simulink model "GroundRelayOC"  (R2025a)
settings: Solver=ode23tb  StartTime=0.0  StopTime=1  RelTol=1e-3  EnableMultiTasking=on
libraries: spsThreePhaseSeriesRLCLoadLib x5, spsDistributedParametersLineLib x5, spsThreePhaseVIMeasurementLib x2, spsRMSLib x1, spsThreePhaseBreakerLib x1, spsThreePhaseFaultLib x1, spsThreePhaseSourceLib x1, spspowerguiLib x1
settings Model: Creator=Rodney Tan  LastModifiedBy=Sanny
settings SolverCC: AlgebraicLoopSolver=TrustRegion
settings DataIOCC: LimitDataPoints=on  SaveFormat=Array  ReturnWorkspaceOutputs=off
settings OptimizationCC: LifeSpan=inf
settings DebuggingCC: UnconnectedInputMsg=warning  UnconnectedOutputMsg=warning  UnconnectedLineMsg=warning  SFUnexpectedBacktrackingDiag=warning  SFNoUnconditionalDefaultTransitionDiag=warning  SFExecutionAtInitializationDiag=none  ArithmeticOperatorsInVariantConditions=warning
settings HardwareCC: ProdBitPerPointer=32.0  ProdBitPerSizeT=32.0  ProdBitPerPtrDiffT=32.0  ProdLargestAtomicFloat=None  ProdIntDivRoundTo=Undefined  ProdEndianess=Unspecified  ProdWordSize=32.0  ProdHWDeviceType=32-bit Generic
settings ModelReferenceCC: EnableRefExpFcnMdlSchedulingChecks=on  PropagateSignalLabelsOutOfModel=off
settings SFSimCC: SimUseLocalCustomCode=off  CustomCodeUndefinedFunction=UseInterfaceOnly
settings RTWCC: RTWUseLocalCustomCode=off  GPUComputeCapability=3.5
settings CodeAppCC: StateflowObjectComments=on
settings GRTTargetCC: TargetLangStandard=C89/C90 (ANSI)
settings ConfigComp: CovMetricSettings=dw  CovSaveCumulativeToWorkspaceVar=on  CovSaveSingleToWorkspaceVar=on  CovExternalEMLEnable=off
settings SimscapeCC: SimscapeNormalizeSystem=off

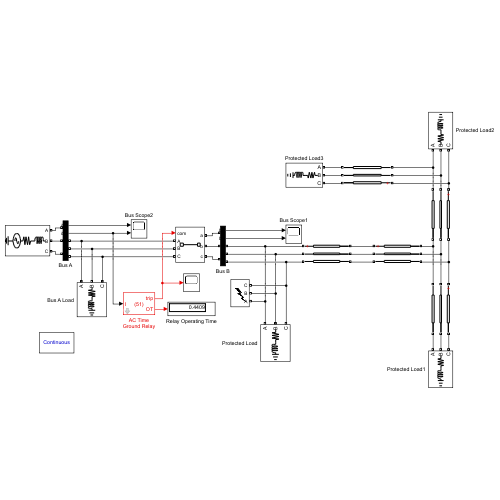
[thumbnail: Simulink's stored preview of the top-level diagram]
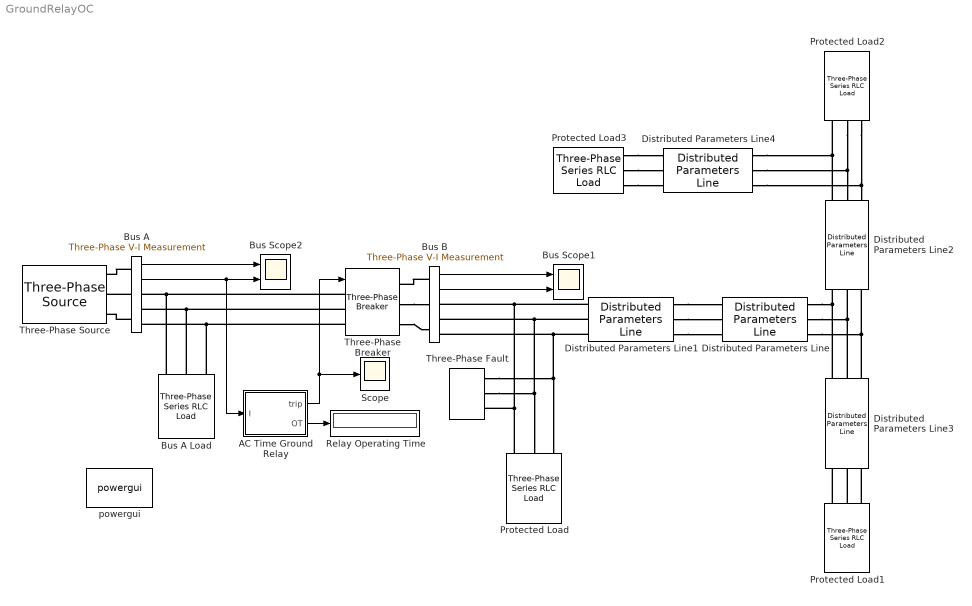
== system GroundRelayOC ==
  AC Time Ground Relay : Subsystem  mask(AC Time Ground Relay Block){tcpopup=IEC Standard Inverse, k=0.14, alpha=0.02, B=0, PS=100%, TMS=0.1, TDS=0.1, CTpri=300, CTsec=5, Freq=50, RMSInit=0}
      mask prompts: tcpopup "Trip Characteristic"; PS "Plug Setting (PS) / Low-set (I >)"; TMS "Time Multiplier Setting (TMS)"; TDS "Time Delay Setting (TDS) in sec"; CTpri "Current Transformer Primary (A)"; CTsec "Current Transformer Secondary (A)"; Freq "Fundamental frequency (Hz):"; RMSInit "Initial RMS value:"
      mask help:
      | AC Time Ground Relay Block developed
      |
      | AC Time Ground  Relay (ANSI/IEEE C37.2 device number 51) that operates when the current exceeds a predetermined value.
      |
      | This relay operates with either a Definite Minimum Time (DMT) or Inverse Definite Minimum Time (IDMT) characteristic.
      |
      | This relay support both IEC 60255 Standard and IEEE Standard C37.112-1996 IDMT trip characteristic.
      mask Help:
      | <b><u>Block Setting</u></b>
      | <b>Trip Characteristic</b>
      | Relay operation mode selection of Definite Minimum Time (DMT), IEC 60255 Standard or IEEE Standard C37.112-1996 Inverse Definite Minimum Time (IDMT).
      | 
      | <b>Plug-Setting(PS) / Low-set (I >)</b>
      | Specify relay pick-up current based on current transformer rating ranging from 25% to 200% with 25% step interval.
      | 
      | <b>Time Multiplier Setting (TMS)</b>
      | Specify time delay multiplier ranging from 0.05 to 1.0 for IDMT relay operation. This setting will be disabled DMT relay operation mode.
      | 
      | <b>Plot Curve Button</b>
      | Plot current Inverse Definite Minimum Time trip curve.
      | 
      | <b>Time Delay Setting (TDS)</b>
      | Specify time delay ranging from 0.05sec to 99sec for Definite Minimum Time relay operation. This setting will be disabled in IDMT relay operation mode.
      | 
      | <b>Current Transformer Primary (A)</b>
      | Specify current transformer primary in Ampere.
      | 
      | <b>Current Transformer Secondary (A)</b>
      | Specify current transformer secondary in Ampere.
      | 
      | <b>Fundamental Frequency (Hz)</b>
      | Specify the RMS current measurement fundamental frequency, in hertz, of the input signal.
      | 
      | <b>Initial RMS Value</b>
      | Specify the RMS current measurement initial RMS value of the output signal.
      | 
      | <b><u>Block Input Output</u></b>
      | <b>I</b>
      | Current input to the AC time overcurrent relay
      | 
      | <b>trip</b>
      | Trip control signal output (1-0), commonly connected to circuit breaker
      | 
      | <b>OT</b>
      | Relay operating time output
      mask TypeOptions tcpopup: Definite Minimum Time | IEC Standard Inverse | IEC Very Inverse | IEC Long Time Inverse | IEC Extremely Inverse | IEC Ultra Inverse | IEEE Moderately Inverse | IEEE Very Inverse | IEEE Extremely Inverse
      mask Callback tcpopup:
      | switch(get_param(gcb,'tcpopup'))
      |     case 'IEC Standard Inverse'
      |         set_param(gcb,'k','0.14');
      |         set_param(gcb,'alpha','0.02');
      |         set_param(gcb,'B','0');
      |         set_param(gcb,'MaskEnables',{'on','off','off','off',...
      |                   'on','on','off','on','on','on','on'});
      |     case 'IEC Very Inverse'
      |         set_param(gcb,'k','13.5');
      |         set_param(gcb,'alpha','1');
      |         set_param(gcb,'B','0');
      |         set_param(gcb,'MaskEnables',{'on','off','off','off',...
      |                   'on','on','off','on','on','on','on'});
      |     case 'IEC Long Time Inverse'
      |         set_param(gcb,'k','120');
      |         set_param(gcb,'alpha','1');
      |         set_param(gcb,'B','0');
      |         set_param(gcb,'MaskEnables',{'on','off','off','off',...
      |                   'on','on','off','on','on','on','on'});
      |     case 'IEC Extremely Inverse'
      |         set_param(gcb,'k','80');
      |         set_param(gcb,'alpha','2');
      |         set_param(gcb,'B','0');
      |         set_param(gcb,'MaskEnables',{'on','off','off','off',...
      |                   'on','on','off','on','on','on','on'});
      |     case 'IEC Ultra Inverse'
      |         set_param(gcb,'k','315.2');
      |         set_param(gcb,'alpha','2.5');
      |         set_param(gcb,'B','0');
      |         set_param(gcb,'MaskEnables',{'on','off','off','off',...
      |                   'on','on','off','on','on','on','on'});
      |     case 'IEEE Moderately Inverse'
      |         set_param(gcb,'k','0.0515');
      |         set_param(gcb,'alpha','0.02');
      |         set_param(gcb,'B','0.114');
      |         set_param(gcb,'MaskEnables',{'on','off','off','off',...
      |                   'on','on','off','on','on','on','on'});
      |     case 'IEEE Very Inverse'
      |         set_param(gcb,'k','19.61');
      |         set_param(gcb,'alpha','2');
      |         set_param(gcb,'B','0.491');
      |         set_param(gcb,'MaskEnables',{'on','off','off','off',...
      |                   'on','on','off','on','on','on','on'});
      |     case 'IEEE Extremely Inverse'
      |         set_param(gcb,'k','28.2');
      |         set_param(gcb,'alpha','2');
      |         set_param(gcb,'B','0.1217');
      |         set_param(gcb,'MaskEnables',{'on','off','off','off',...
      |                   'on','on','off','on','on','on','on'});
      |     otherwise
      |         set_param(gcb,'k','0');
      |         set_param(gcb,'MaskEnables',{'on','off','off','off',...
      |                   'on','off','on','on','on','on','on'});
      | end
      mask TypeOptions PS: 25% | 50% | 75% | 100% | 125% | 150% | 175% | 200%
      mask TypeOptions TMS: 0.05 | 0.1 | 0.15 | 0.2 | 0.25 | 0.3 | 0.35 | 0.4 | 0.45 | 0.5 | 0.55 | 0.6 | 0.65 | 0.7 | 0.75 | 0.8 | 0.85 | 0.9 | 0.95 | 1.0
      mask Callback TDS:
      | TDS = str2double(get_param(gcb,'TDS'));
      | if (TDS > 99)||(TDS < 0.05)||isnan(TDS)
      |     msgbox('TDS must be in the range of 0.05-99 sec',...
      |     'Invalid Value !','error');
      |     set_param(gcb,'TDS','0.1');
      | end
      mask TypeOptions Freq: Irms/Freq
      mask TypeOptions RMSInit: Irms/RMSInit
      mask DialogControl Container2 Prompt: Relay Setting
      mask DialogControl plotbutton Prompt: Plot Curve
      mask DialogControl plotbutton Callback:
      | % Plotting IDMT Curve
      | TMS = str2num(get_param(gcb,'TMS'));
      | k = str2num(get_param(gcb,'k'));
      | alpha = str2num(get_param(gcb,'alpha'));
      | B = str2num(get_param(gcb,'B'));
      | I = 1:20;
      | td = ((k./((I.^alpha)-1))+B)*TMS;
      | loglog(td);
      | set(gcf, 'Position', [200 150 300 500]);
      | switch(get_param(gcb,'tcpopup'))
      |     case 'IEC Standard Inverse'
      |         title('IEC Standard Inverse');
      |         set(gca, 'YTick', (1:10));
      |         ylim([0.1 10]);
      |     case 'IEC Very Inverse'
      |         title('IEC Very Inverse');
      |         set(gca, 'YTick', (1:2:15));
      |         ylim([0.01 15]);
      |     case 'IEC Long Time Inverse'
      |         title('IEC Long Time Inverse');
      |         set(gca, 'YTick', (0:20:120));
      |         ylim([0.1 120]);
      |     case 'IEC Extremely Inverse'
      |         title('IEC Extremely Inverse');
      |         set(gca, 'YTick', (0:5:30));
      |         ylim([0.01 30]);
      |     case 'IEC Ultra Inverse'
      |         title('IEC Ultra Inverse');
      |         set(gca, 'YTick', (0:20:100));
      |         ylim([0.01 100]);
      |     case 'IEEE Moderately Inverse'
      |         title('IEEE Moderately Inverse');
      |         set(gca, 'YTick', (1:5));
      |         ylim([0.01 5]);
      |     case 'IEEE Very Inverse'
      |         title('IEEE Very Inverse');
      |         set(gca, 'YTick', (1:10));
      |         ylim([0.01 10]);
      |     case 'IEEE Extremely Inverse'
      |         title('IEEE Extremely Inverse');
      |         set(gca, 'YTick', (1:10));
      |         ylim([0.01 10]);
      | end
      | 
      | set(gca, 'XTick', [1:10 20]);
      | xlim([1 30]);
      | xlabel('Current (Multiples of Plug Setting)');
      | ylabel('Operating Time (sec)');
      | grid on;
      mask DialogControl Container3 Prompt: Current Transformer Setting
      mask DialogControl RMS Prompt: RMS Current Measurement
      mask Display:
      | disp('(51)');
      | port_label('input', 1, 'I');
      | port_label('output', 1, 'trip');
      | port_label('output', 2, 'OT');
  Bus A : spsThreePhaseVIMeasurementLib/Three-Phase V-I Measurement  VoltageMeasurement=phase-to-ground  SetLabelV=off  LabelV=Vabc  Vpu=off  VpuLL=off  CurrentMeasurement=yes  SetLabelI=off  LabelI=Iabc  Ipu=off  Pbase=100e6  Vbase=500e3  OutputType=Complex  PhasorSimulation=off  PSBequivalent=0
  Bus A Load : spsThreePhaseSeriesRLCLoadLib/Three-Phase Series RLC Load  LConnTagsString=A|B|C  Configuration=Y (grounded)  NominalVoltage=400  Vabc=[1e3 1e3 1e3]  Vabcp=[1e3 1e3 1e3]  NominalFrequency=50  UnbalancedPower=off  ActivePower=100e3  InductivePower=1000  CapacitivePower=0  Pabc=[10e3 9e3 11e3]  QLabc=[100 90 110]  QCabc=[100 90 110]  Pabcp=[10e3 9e3 11e3]  QLabcp=[100 90 110]  QCabcp=[100 90 110]  Measurements=None  LoadType=constant Z
  Bus B : spsThreePhaseVIMeasurementLib/Three-Phase V-I Measurement  VoltageMeasurement=phase-to-ground  SetLabelV=off  LabelV=Vabc  Vpu=off  VpuLL=off  CurrentMeasurement=yes  SetLabelI=off  LabelI=Iabc  Ipu=off  Pbase=100e6  Vbase=500e3  OutputType=Complex  PhasorSimulation=off  PSBequivalent=0
  Bus Scope1 : Scope  NumInputPorts=2
      settings: Title=Bus B Current Profile  ShowGrid=off  ActiveDisplayYMinimum=-2533.58175  ActiveDisplayYMaximum=3369.6826  YLabel=Current (A)  DataLoggingSaveFormat=Array
  Bus Scope2 : Scope  NumInputPorts=2
      settings: Title=Bus A Current Profile  ShowGrid=off  ActiveDisplayYMinimum=-3316.7768762510213  ActiveDisplayYMaximum=3723.0047575859285  YLabel=Current (A)  DataLoggingSaveFormat=Array
  Distributed Parameters Line : spsDistributedParametersLineLib/Distributed Parameters Line  Phases=3  Length=100  Frequency=60  Resistance=[0.01273 0.3864]  Inductance="[0.9337e-3  4.1264e-3]"  Capacitance=[12.74e-9 7.751e-9]  x1=[1.91730079564317e-11 400.864028866089 400.864028866057;314.159265358979 314.159265358979 314.159265358979;-1.26095069546775 0.22104226848999 -1.34975405830491]  x2=[2.10404277961572e-11 418.154854663515 418.154854663482;314.159265358979 314.159265358979 314.159265358979;-1.25793304118418 0.218562240810716 -1.35223408598418]  x3=[3.3168484674381e-14 1.61146629060892 1.6114662906088;314.159265358979 314.159265358979 314.159265358979;-1.67750735657674 -0.207558438130243 -1.77835476492514]  x4=[2.86533303244721e-14 1.6281634973106 1.62816349731047;314.159265358979 314.159265358979 314.159265358979;-0.811737549604632 0.534619710597266 -1.03617661619763]  x5=0.000565541566995742  V1=[1.917e-11 400.9 400.9;314.2 314.2 314.2;-1.261 0.221 -1.35]  V2=[2.104e-11 418.2 418.2;314.2 314.2 314.2;-1.258 0.2186 -1.352]  I1=[3.317e-14 1.611 1.611;314.2 314.2 314.2;-1.678 -0.2076 -1.778]  I2=[2.865e-14 1.628 1.628;314.2 314.2 314.2;-0.8117 0.5346 -1.036]  nHarmo=1  Measurements=None  Decoupling=off  VsMag0=0  VrMag0=0  VsAngle0=0  VrAngle0=0  IsMag0=0  IrMag0=0  IsAngle0=0  IrAngle0=0
      settings: LibrarySourceBlock=sps_lib/Power Grid Elements/Distributed Parameters Line
  Distributed Parameters Line1 : spsDistributedParametersLineLib/Distributed Parameters Line  Phases=3  Length=100  Frequency=60  Resistance=[0.01273 0.3864]  Inductance="[0.9337e-3  4.1264e-3]"  Capacitance=[12.74e-9 7.751e-9]  x1=[1.66634921443281e-11 378.874881999354 378.874881999324;314.159265358979 314.159265358979 314.159265358979;-1.25735531670556 0.22431743741207 -1.34647888938283]  x2=[1.91981231328159e-11 400.864028866089 400.864028866057;314.159265358979 314.159265358979 314.159265358979;-1.26164418272018 0.22104226848999 -1.34975405830491]  x3=[3.2858812901172e-14 1.61004045973489 1.61004045973477;314.159265358979 314.159265358979 314.159265358979;-1.86057715853467 -0.314042437625186 -1.88483876442008]  x4=[2.74177794533837e-14 1.62934933429943 1.62934933429929;314.159265358979 314.159265358979 314.159265358979;-0.630736116597079 0.644633634719405 -0.926162692075487]  x5=0.000565541566995742  V1=[1.666e-11 378.9 378.9;314.2 314.2 314.2;-1.257 0.2243 -1.346]  V2=[1.92e-11 400.9 400.9;314.2 314.2 314.2;-1.262 0.221 -1.35]  I1=[3.286e-14 1.61 1.61;314.2 314.2 314.2;-1.861 -0.314 -1.885]  I2=[2.742e-14 1.629 1.629;314.2 314.2 314.2;-0.6307 0.6446 -0.9262]  nHarmo=1  Measurements=None  Decoupling=off  VsMag0=0  VrMag0=0  VsAngle0=0  VrAngle0=0  IsMag0=0  IrMag0=0  IsAngle0=0  IrAngle0=0
      settings: LibrarySourceBlock=sps_lib/Power Grid Elements/Distributed Parameters Line
  Distributed Parameters Line2 : spsDistributedParametersLineLib/Distributed Parameters Line  Phases=3  Length=100  Frequency=60  Resistance=[0.01273 0.3864]  Inductance="[0.9337e-3  4.1264e-3]"  Capacitance=[12.74e-9 7.751e-9]  x1=[2.2104307302334e-11 425.635026191159 425.635026191177;314.159265358979 314.159265358979 314.159265358979;-1.27734341959448 1.264607271327 2.83540359812197]  x2=[2.10312439975579e-11 418.15485466349 418.154854663507;314.159265358979 314.159265358979 314.159265358979;-1.2573167080909 1.26575979200728 2.83655611880225]  x3=[3.12380835243649e-14 1.58125065905922 1.58125065905928;314.159265358979 314.159265358979 314.159265358979;-1.05804899780135 1.37238132652106 2.94317765331603]  x4=[3.00220202002779e-14 1.57045481453233 1.5704548145324;314.159265358979 314.159265358979 314.159265358979;-1.58568603341573 1.04837602697857 2.61917235377353]  x5=0.000565541566995742  V1=[2.21e-11 425.6 425.6;314.2 314.2 314.2;-1.277 1.265 2.835]  V2=[2.103e-11 418.2 418.2;314.2 314.2 314.2;-1.257 1.266 2.837]  I1=[3.124e-14 1.581 1.581;314.2 314.2 314.2;-1.058 1.372 2.943]  I2=[3.002e-14 1.57 1.57;314.2 314.2 314.2;-1.586 1.048 2.619]  nHarmo=1  Measurements=None  Decoupling=off  VsMag0=0  VrMag0=0  VsAngle0=0  VrAngle0=0  IsMag0=0  IrMag0=0  IsAngle0=0  IrAngle0=0
      settings: LibrarySourceBlock=sps_lib/Power Grid Elements/Distributed Parameters Line
  Distributed Parameters Line3 : spsDistributedParametersLineLib/Distributed Parameters Line  Phases=3  Length=100  Frequency=60  Resistance=[0.01273 0.3864]  Inductance="[0.9337e-3  4.1264e-3]"  Capacitance=[12.74e-9 7.751e-9]  x1=[2.10187140598747e-11 418.15485466349 418.154854663507;314.159265358979 314.159265358979 314.159265358979;-1.25699782996798 1.26575979200728 2.83655611880225]  x2=[2.12460785323591e-11 420.61040635086 420.610406350877;314.159265358979 314.159265358979 314.159265358979;-1.25968948203942 1.2653207935263 2.83611712032126]  x3=[2.989042365455e-14 1.54558853383228 1.54558853383234;314.159265358979 314.159265358979 314.159265358979;-1.39382361404444 1.15726490876129 2.72806123555627]  x4=[2.93775944398719e-14 1.55083211138511 1.55083211138517;314.159265358979 314.159265358979 314.159265358979;-1.27041654471723 1.26515168163053 2.83594800842548]  x5=0.000565541566995742  V1=[2.102e-11 418.2 418.2;314.2 314.2 314.2;-1.257 1.266 2.837]  V2=[2.125e-11 420.6 420.6;314.2 314.2 314.2;-1.26 1.265 2.836]  I1=[2.989e-14 1.546 1.546;314.2 314.2 314.2;-1.394 1.157 2.728]  I2=[2.938e-14 1.551 1.551;314.2 314.2 314.2;-1.27 1.265 2.836]  nHarmo=1  Measurements=None  Decoupling=off  VsMag0=0  VrMag0=0  VsAngle0=0  VrAngle0=0  IsMag0=0  IrMag0=0  IsAngle0=0  IrAngle0=0
      settings: LibrarySourceBlock=sps_lib/Power Grid Elements/Distributed Parameters Line
  Distributed Parameters Line4 : spsDistributedParametersLineLib/Distributed Parameters Line  Phases=3  Length=100  Frequency=60  Resistance=[0.01273 0.3864]  Inductance="[0.9337e-3  4.1264e-3]"  Capacitance=[12.74e-9 7.751e-9]  x1=[2.2104307302334e-11 425.635026191159 425.635026191177;314.159265358979 314.159265358979 314.159265358979;-1.27734341959448 1.264607271327 2.83540359812197]  x2=[2.25389935028865e-11 428.134504064276 428.134504064294;314.159265358979 314.159265358979 314.159265358979;-1.24730822726929 1.26416827284602 2.83496459964099]  x3=[3.64008136046968e-14 1.57323682540495 1.57323682540501;314.159265358979 314.159265358979 314.159265358979;-1.37126949269881 1.15611238808101 2.72690871487598]  x4=[2.59932696411518e-14 1.57857420280029 1.57857420280036;314.159265358979 314.159265358979 314.159265358979;-1.2685412090439 1.26399916095025 2.83479548774522]  x5=0.000565541566995742  V1=[2.21e-11 425.6 425.6;314.2 314.2 314.2;-1.277 1.265 2.835]  V2=[2.254e-11 428.1 428.1;314.2 314.2 314.2;-1.247 1.264 2.835]  I1=[3.64e-14 1.573 1.573;314.2 314.2 314.2;-1.371 1.156 2.727]  I2=[2.599e-14 1.579 1.579;314.2 314.2 314.2;-1.269 1.264 2.835]  nHarmo=1  Measurements=None  Decoupling=off  VsMag0=0  VrMag0=0  VsAngle0=0  VrAngle0=0  IsMag0=0  IrMag0=0  IsAngle0=0  IrAngle0=0
      settings: LibrarySourceBlock=sps_lib/Power Grid Elements/Distributed Parameters Line
  Protected Load : spsThreePhaseSeriesRLCLoadLib/Three-Phase Series RLC Load  LConnTagsString=A|B|C  Configuration=Y (grounded)  NominalVoltage=400  Vabc=[1e3 1e3 1e3]  Vabcp=[1e3 1e3 1e3]  NominalFrequency=50  UnbalancedPower=off  ActivePower=100e3  InductivePower=1000  CapacitivePower=0  Pabc=[10e3 9e3 11e3]  QLabc=[100 90 110]  QCabc=[100 90 110]  Pabcp=[10e3 9e3 11e3]  QLabcp=[100 90 110]  QCabcp=[100 90 110]  Measurements=None  LoadType=constant Z
  Protected Load1 : spsThreePhaseSeriesRLCLoadLib/Three-Phase Series RLC Load  LConnTagsString=A|B|C  Configuration=Y (grounded)  NominalVoltage=400  Vabc=[1e3 1e3 1e3]  Vabcp=[1e3 1e3 1e3]  NominalFrequency=50  UnbalancedPower=off  ActivePower=1  InductivePower=.1  CapacitivePower=0  Pabc=[10e3 9e3 11e3]  QLabc=[100 90 110]  QCabc=[100 90 110]  Pabcp=[10e3 9e3 11e3]  QLabcp=[100 90 110]  QCabcp=[100 90 110]  Measurements=None  LoadType=constant Z
  Protected Load2 : spsThreePhaseSeriesRLCLoadLib/Three-Phase Series RLC Load  LConnTagsString=A|B|C  Configuration=Y (grounded)  NominalVoltage=400  Vabc=[1e3 1e3 1e3]  Vabcp=[1e3 1e3 1e3]  NominalFrequency=50  UnbalancedPower=off  ActivePower=1  InductivePower=.1  CapacitivePower=0  Pabc=[10e3 9e3 11e3]  QLabc=[100 90 110]  QCabc=[100 90 110]  Pabcp=[10e3 9e3 11e3]  QLabcp=[100 90 110]  QCabcp=[100 90 110]  Measurements=None  LoadType=constant Z
  Protected Load3 : spsThreePhaseSeriesRLCLoadLib/Three-Phase Series RLC Load  LConnTagsString=A|B|C  Configuration=Y (grounded)  NominalVoltage=400  Vabc=[1e3 1e3 1e3]  Vabcp=[1e3 1e3 1e3]  NominalFrequency=50  UnbalancedPower=off  ActivePower=1  InductivePower=.1  CapacitivePower=0  Pabc=[10e3 9e3 11e3]  QLabc=[100 90 110]  QCabc=[100 90 110]  Pabcp=[10e3 9e3 11e3]  QLabcp=[100 90 110]  QCabcp=[100 90 110]  Measurements=None  LoadType=constant Z
  Relay Operating Time : Display
  Scope : Scope
      settings: ActiveDisplayYMinimum=-0.12499999999999997  ActiveDisplayYMaximum=1.125  DataLoggingVariableName=ScopeData3  DataLoggingSaveFormat=Array
  Three-Phase Breaker : spsThreePhaseBreakerLib/Three-Phase Breaker  InitialState=closed  SwitchA=on  SwitchB=on  SwitchC=on  SwitchTimes="[1/60  5/60]"  External=on  BreakerResistance=0.01  SnubberResistance=1e6  SnubberCapacitance=inf  Measurements=None
  Three-Phase Fault : spsThreePhaseFaultLib/Three-Phase Fault  InitialStates=0  FaultA=on  FaultB=on  FaultC=on  GroundFault=on  SwitchTimes=0.1  External=off  SwitchStatus=NaN  FaultResistance=0.001  GroundResistance=0.01  SnubberResistance=1e6  SnubberCapacitance=inf  Measurements=None
  Three-Phase Source : spsThreePhaseSourceLib/Three-Phase Source  InternalConnection=Yg  VoltagePhases=off  Voltage=400  PhaseAngle=0  Voltage_phases=[25e3 25e3 25e3]/sqrt(3)  PhaseAngles_phases=[0 -120 +120]  Frequency=50  NonIdealSource=on  SpecifyImpedance=on  Resistance=0.8929  Inductance=16.58e-3  ShortCircuitLevel=1e6  BaseVoltage=400  XRratio=7  BusType=swing  Pref=0  Qref=0  Prefabc=[10e3, 10e3, 10e3]  Qrefabc=[0, 0, 0]  Qmin=-inf  Qmax=inf
  powergui : spspowerguiLib/powergui  Priority=1  SimulationMode=Continuous  SampleTime=50e-6  frequency=60  Iterations=50  frequencyindice=50  Pbase=100e6  ErrMax=1e-4  UnitsV=kV  UnitsW=MW  buscounter=0  FunctionMessages=off  echomessages=off  EnableUseOfTLC=off  CurrentSourceSwitches=off  DisableSnubberDevices=on  DisableRonSwitches=off  DisableVfSwitches=off  DisplayEquations=off  AutomaticDiscreteSolvers=off  SolverType=Tustin/Backward Euler (TBE)  Interpol=off  ExternalGateDelay=off  methode=off  Ts=100  x0status=blocks  SPID=on  SwTol=0  HookPort=off  NonlinearTolerance=1e-4  nMaxIteration=100  ContinueOnMaxIteration=off  RestoreLinks=warning  ResistiveCurrentMeasurement=off  Frange=[0:2:500]  Ylog=off  Xlog=on  ShowGrid=off  save=off  variable=ZData  structure=0  ZoomFFT=off  StartTime=0.0  cycles=1  DisplayStyle=1  fundamental=60  FreqAxis=off  MaxFrequency=1000  frequencyindicesteady=1  RmsSteady=1  display=off
  wires:
  Bus A/2 -> Bus Scope2/2, AC Time Ground Relay/1(I)
  AC Time Ground Relay/1(trip) -> Three-Phase Breaker/1, Scope/1
  Bus A/1 -> Bus Scope2/1
  Bus B/1 -> Bus Scope1/1
  Bus B/2 -> Bus Scope1/2
  AC Time Ground Relay/2(OT) -> Relay Operating Time/1
  connections:
  Bus A/LConn1 -- Three-Phase Source/RConn1
  Three-Phase Breaker/LConn2 -- Bus A Load/LConn2 -- Bus A/RConn2
  Three-Phase Breaker/LConn1 -- Bus A Load/LConn1 -- Bus A/RConn1
  Bus A/LConn2 -- Three-Phase Source/RConn2
  Bus A/LConn3 -- Three-Phase Source/RConn3
  Three-Phase Breaker/LConn3 -- Bus A Load/LConn3 -- Bus A/RConn3
  Three-Phase Breaker/RConn2 -- Bus B/LConn2
  Bus B/LConn1 -- Three-Phase Breaker/RConn1
  Three-Phase Breaker/RConn3 -- Bus B/LConn3
  Three-Phase Fault/LConn2 -- Bus B/RConn2 -- Distributed Parameters Line1/LConn2 -- Protected Load/LConn2
  Three-Phase Fault/LConn3 -- Protected Load/LConn3 -- Bus B/RConn3 -- Distributed Parameters Line1/LConn3
  Protected Load/LConn1 -- Three-Phase Fault/LConn1 -- Bus B/RConn1 -- Distributed Parameters Line1/LConn1
  Distributed Parameters Line1/RConn3 -- Distributed Parameters Line/LConn3
  Distributed Parameters Line1/RConn2 -- Distributed Parameters Line/LConn2
  Distributed Parameters Line/RConn1 -- Distributed Parameters Line2/RConn3 -- Distributed Parameters Line3/LConn3
  Distributed Parameters Line/RConn2 -- Distributed Parameters Line3/LConn2 -- Distributed Parameters Line2/RConn2
  Distributed Parameters Line/RConn3 -- Distributed Parameters Line3/LConn1 -- Distributed Parameters Line2/RConn1
  Protected Load1/LConn3 -- Distributed Parameters Line3/RConn1
  Protected Load1/LConn2 -- Distributed Parameters Line3/RConn2
  Protected Load1/LConn1 -- Distributed Parameters Line3/RConn3
  Protected Load2/LConn3 -- Distributed Parameters Line4/LConn1 -- Distributed Parameters Line2/LConn1
  Protected Load2/LConn2 -- Distributed Parameters Line4/LConn2 -- Distributed Parameters Line2/LConn2
  Distributed Parameters Line2/LConn3 -- Protected Load2/LConn1 -- Distributed Parameters Line4/LConn3
  Protected Load3/LConn3 -- Distributed Parameters Line4/RConn1
  Protected Load3/LConn1 -- Distributed Parameters Line4/RConn3
  Protected Load3/LConn2 -- Distributed Parameters Line4/RConn2
  Distributed Parameters Line1/RConn1 -- Distributed Parameters Line/LConn1

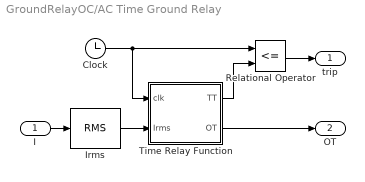
== system GroundRelayOC/AC Time Ground Relay ==
  I : Inport
  Clock : Clock
  Irms : spsRMSLib/RMS  TrueRMS=on  Freq=Freq  RMSInit=RMSInit  Ts=0
  Relational Operator : RelationalOperator  Operator=<=  OutDataTypeStr=boolean  InputSameDT=off
  Time Relay Function : MATLAB Function  TreatAsAtomicUnit=on
  trip : Outport  VectorParamsAs1DForOutWhenUnconnected=off
  OT : Outport  Port=2  VectorParamsAs1DForOutWhenUnconnected=off
  wires:
  Clock/1 -> Relational Operator/1, Time Relay Function/1(clk)
  Irms/1 -> Time Relay Function/2(Irms)
  Time Relay Function/1(TT) -> Relational Operator/2
  Time Relay Function/2(OT) -> OT/1
  Relational Operator/1 -> trip/1
  I/1 -> Irms/1

== matlab function GroundRelayOC/AC Time Ground Relay/Time Relay Function ==
  settings: updateMethod=DISCRETE
  data: TT output; clk input; Irms input; CTpri parameter; CTsec parameter; PS parameter; OT output; TMS parameter; k parameter; alpha parameter; B parameter; TDS parameter
function [TT, OT] = fcn(clk,Irms,CTpri,CTsec,PS,TMS,k,alpha,B,TDS)

persistent RelayState TripTime OperatingTime PickupTime

if isempty(RelayState)
    RelayState = 0;
    TripTime = inf;
    OperatingTime = inf;
    PickupTime = 0;
end

CT = max(Irms/(CTpri/CTsec));
Pickup = (PS*0.25)*CTsec;

if (RelayState == 0)&&(CT > Pickup)
    PickupTime = clk;
    RelayState = 1;
end

if (RelayState == 1)&&(clk>(PickupTime+0.02)) % Wait for 20ms fault current rise time
    if k == 0
        OperatingTime = TDS;
    else
        PMS = CT/Pickup;                          % Calculate Plug Multiplier Setting
        OperatingTime = ((k/((PMS^alpha)-1))+B)*(TMS*0.05); % Determine Definite Inverse Minimum Time
    end
    TripTime = PickupTime + OperatingTime;
    RelayState = 2;
end

TT = TripTime;
OT = OperatingTime;
